simulink model "CustomBaseControl"  (R2022a)
settings: Solver=VariableStepAuto  StartTime=0.0  StopTime=20  RelTol=1e-3
values from neighbouring files (symbols this model uses):
  den = [1 2 1]    [Process.m]
  DERIVATIVE_GAIN = 0    [Process.m]
  INTEGRAL_GAIN = zn_parameters.Kp / zn_parameters.Ti    [Process.m]
  num = 2    [Process.m]
settings Model: Creator=lucas  LastModifiedBy=lucas

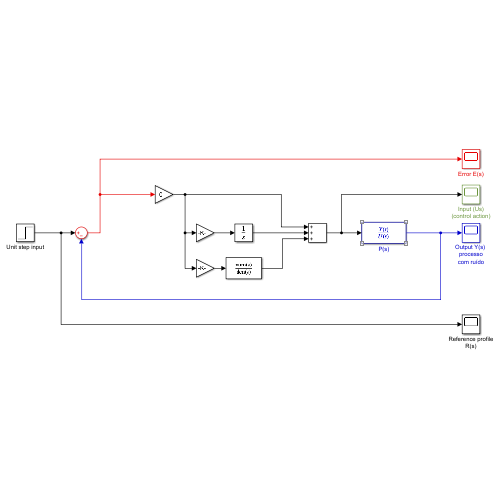
[thumbnail: Simulink's stored preview of the top-level diagram]
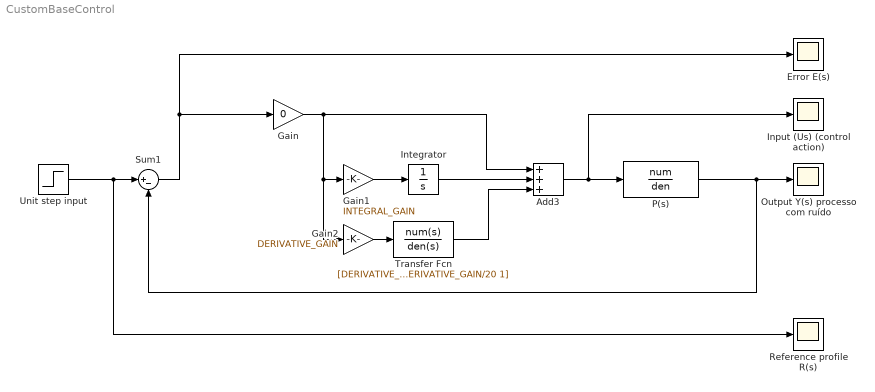
== system CustomBaseControl ==
  Add3 : Sum  Inputs=+++
  Error E(s) : Scope
  Gain : Gain  Gain=0
  Gain1 : Gain  Gain=INTEGRAL_GAIN
  Gain2 : Gain  Gain=DERIVATIVE_GAIN
  Input (Us) (control action) : Scope
  Integrator : Integrator
  Output Y(s) processo com ruído : Scope
  P(s) : TransferFcn  Numerator=num  Denominator=den
  Reference profile R(s) : Scope
  Sum1 : Sum  Inputs=|+-
  Transfer Fcn : TransferFcn  Numerator=[DERIVATIVE_GAIN 0]  Denominator=[DERIVATIVE_GAIN/20 1]
  Unit step input : Step  Time=5  SampleTime=0
  wires:
  Sum1/1 -> Gain/1, Error E(s)/1
  Unit step input/1 -> Sum1/1, Reference profile R(s)/1
  P(s)/1 -> Sum1/2, Output Y(s) processo com ruído/1
  Gain/1 -> Add3/1, Gain2/1, Gain1/1
  Gain1/1 -> Integrator/1
  Gain2/1 -> Transfer Fcn/1
  Integrator/1 -> Add3/2
  Transfer Fcn/1 -> Add3/3
  Add3/1 -> P(s)/1, Input (Us) (control action)/1
